simulink model "modelo2"  (Simulink 8.5)
settings: Solver=ode45  StartTime=0.0  StopTime=3600  RelTol=1e-3
values from neighbouring files (symbols this model uses):
  Hz = 10    [modelo_controlador_analisis.m]
  T = 0.02    [modelo_controlador_analisis.m]
libraries: simulink x1
settings Model: Creator=n421  LastModifiedBy=ARTURO  CovModelRefEnable=off
settings DataIOCC: SaveFormat=Dataset  SignalLoggingSaveFormat=Dataset
settings OptimizationCC: ExpressionDepthLimit=128
settings DebuggingCC: UnderspecifiedInitializationDetection=Simplified  MergeDetectMultiDrivingBlocksExec=error  FcnCallInpInsideContextMsg=EnableAllAsError  StateNameClashWarn=none
settings HardwareCC: ProdBitPerPointer=64  ProdLargestAtomicFloat=Float  ProdIntDivRoundTo=Zero  ProdEndianess=LittleEndian  ProdHWDeviceType=Specified
settings GRTTargetCC: GeneratePreprocessorConditionals=Use local settings  CombineOutputUpdateFcns=on  GRTInterface=off

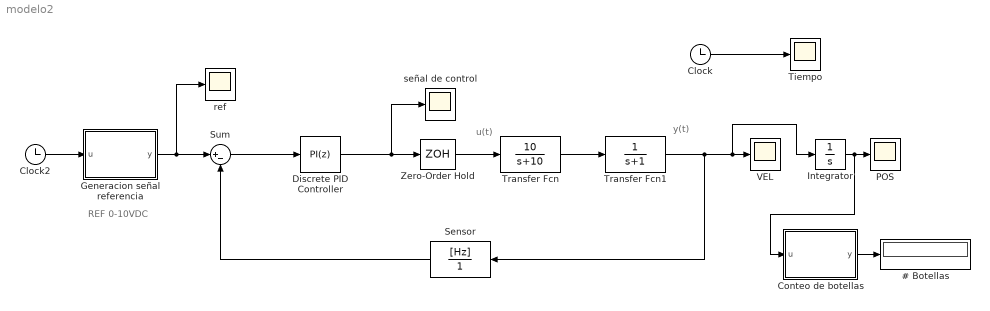
== system modelo2 ==
  note: y(t)
  note: u(t)
  note: REF 0-10VDC
  # Botellas : Display
  Clock : Clock
  Clock2 : Clock
  Conteo de botellas : MATLAB Function  TreatAsAtomicUnit=on
  Discrete PID Controller : simulink/Continuous/PID Controller  Controller=PI  TimeDomain=Discrete-time  SampleTime=T  IntegratorMethod=Trapezoidal  FilterMethod=Forward Euler  Form=Parallel  UseFilter=on  ControllerParametersSource=internal  P=0.8511  I=0.5881  D=0  N=100  InitialConditionSource=internal  InitialConditionForIntegrator=0  InitialConditionForFilter=0  ExternalReset=none  LimitOutput=off  UpperSaturationLimit=inf  LowerSaturationLimit=-inf  LinearizeAsGain=off  AntiWindupMode=none  Kb=1  TrackingMode=off  Kt=1  PParamMin=[]  PParamMax=[]  IParamMin=[]  IParamMax=[]  DParamMin=[]  DParamMax=[]  NParamMin=[]  NParamMax=[]  KbParamMin=[]  KbParamMax=[]  KtParamMin=[]  KtParamMax=[]  POutMin=[]  POutMax=[]  IOutMin=[]  IOutMax=[]  DOutMin=[]  DOutMax=[]  NOutMin=[]  NOutMax=[]  KbOutMin=[]  KbOutMax=[]  KtOutMin=[]  KtOutMax=[]  IntegratorOutMin=[]  IntegratorOutMax=[]  FilterOutMin=[]  FilterOutMax=[]  SumOutMin=[]  SumOutMax=[]  SumI1OutMin=[]  SumI1OutMax=[]  SumI2OutMin=[]  SumI2OutMax=[]  SumI3OutMin=[]  SumI3OutMax=[]  SumDOutMin=[]  SumDOutMax=[]  SaturationOutMin=[]  SaturationOutMax=[]  IntegratorContinuousStateAttributes=''  IntegratorStateMustResolveToSignalObject=off  IntegratorRTWStateStorageClass=Auto  FilterContinuousStateAttributes=''  FilterStateMustResolveToSignalObject=off  FilterRTWStateStorageClass=Auto  DifferentiatorICPrevScaledInput=0  DifferentiatorOutMin=[]  DifferentiatorOutMax=[]
  "Generacion señal referencia " : MATLAB Function  TreatAsAtomicUnit=on
  Integrator : Integrator
  "POS " : Scope
      settings: YMin=11  YMax=13.5  SaveName=pos
  Sensor : DiscreteTransferFcn  Numerator=[Hz]  Denominator=[1]  SampleTime=T
  Sum : Sum  Inputs=|+-
  "Tiempo " : Scope
      settings: YMin=-1.25  YMax=11.25  SaveName=tiempo
  Transfer Fcn : TransferFcn  Numerator=[10]  Denominator=[1 10]
  Transfer Fcn1 : TransferFcn  Denominator=[1 1]
  "VEL " : Scope
      settings: YMin=-0.01406  YMax=0.12652  SaveName=y
  Zero-Order Hold : ZeroOrderHold  SampleTime=T
  ref : Scope
      settings: TimeRange=20  YMin=0  YMax=2.5  SaveName=r
  señal de control : Scope
      settings: YMin=-0.13264  YMax=0.96694  SaveName=u
  wires:
  Transfer Fcn1/1 -> Sensor/1, Integrator/1, "VEL "/1
  Sum/1 -> Discrete PID Controller/1
  Zero-Order Hold/1 -> Transfer Fcn/1
  Transfer Fcn/1 -> Transfer Fcn1/1
  Sensor/1 -> Sum/2
  Discrete PID Controller/1 -> señal de control/1, Zero-Order Hold/1
  Clock/1 -> "Tiempo "/1
  Clock2/1 -> "Generacion señal referencia "/1(u)
  "Generacion señal referencia "/1(y) -> ref/1, Sum/1
  Integrator/1 -> Conteo de botellas/1(u), "POS "/1
  Conteo de botellas/1(y) -> # Botellas/1

== matlab function Conteo de botellas ==
  data: u input double; y output double
function y = fcn(u)

y = u/0.5;

y = 5*ceil(y);

== matlab function Generacion señal referencia  ==
  data: u input double; y output double
function y = fcn(u)
%#codegen
n = floor(u/6);
tt = 4*n;

if tt>0
tll = 2*n; %Tiempo de llenado
else
tll = 0;
end
%2.5*u*(u<1) + 2.5*(u>=1)*(u<2)+(7.5-2.5*u)*(u>=2)*(u<=3)

%y = 2.5*(u-tt)*(u<(tt+1)) + 2.5*(u>=(tt+1))*(u<(tt+2))+(7.5-2.5*(u-tt))*(u>=(tt+2))*(u<=(tt+3))

y = 2.5*(u-tt-tll)*(u<(tt+tll+1)) + 2.5*(u>=(tt+tll+1))*(u<(tt+tll+2))+(7.5-2.5*(u-tt-tll))*(u>=(tt+tll+2))*(u<=(tt+tll+3));
